simulink model "single_phase_thyristor_rect"  (R2022b)
settings: Solver=VariableStepAuto  StartTime=0.0  StopTime=0.04  RelTol=1e-3
undefined symbols (not defined in the file): p
libraries: spsThyristorLib x6, spsVoltageMeasurementLib x4, spsACVoltageSourceLib x3, spsCurrentMeasurementLib x1, spsMeanLib x1, spsSeriesRLCBranchLib x1, spspowerguiLib x1
settings Model: Creator=alman  LastModifiedBy=alman
settings SolverCC: ZeroCrossAlgorithm=Adaptive
settings DebuggingCC: MaskedZcDiagnostic=none  IgnoredZcDiagnostic=none

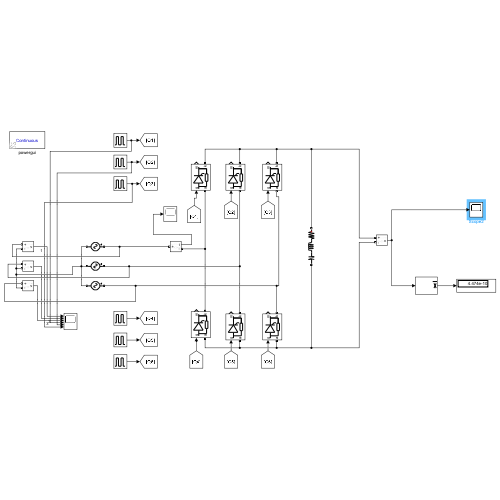
[thumbnail: Simulink's stored preview of the top-level diagram]
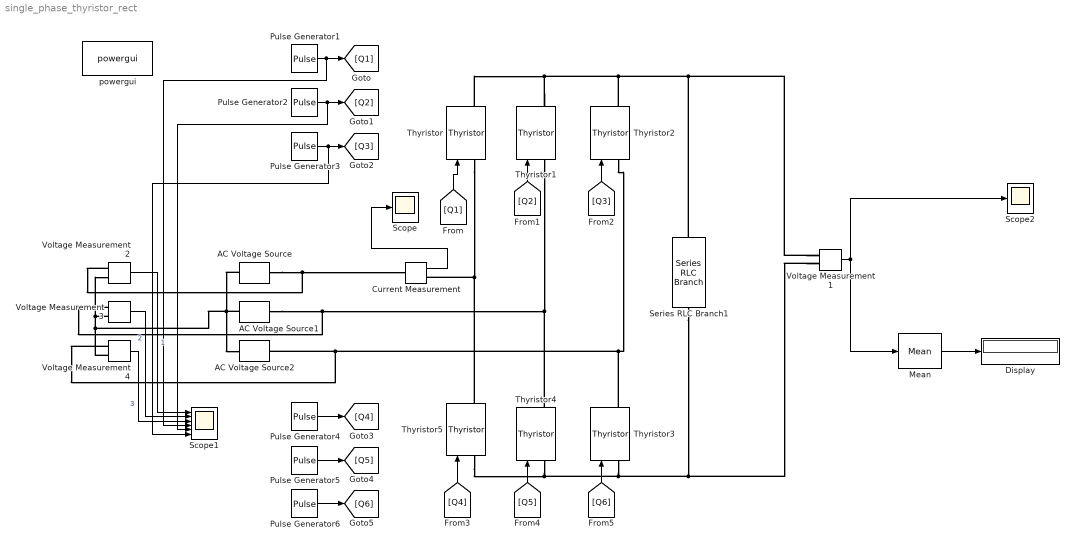
== system single_phase_thyristor_rect ==
  AC Voltage Source : spsACVoltageSourceLib/AC Voltage Source  Amplitude=230*sqrt(2)  Phase=0  Frequency=50  SampleTime=0  Measurements=None  BusType=swing  Pref=10e3  Qref=0  Qmin=-inf  Qmax=+inf
  AC Voltage Source1 : spsACVoltageSourceLib/AC Voltage Source  Amplitude=230*sqrt(2)  Phase=-120  Frequency=50  SampleTime=0  Measurements=None  BusType=swing  Pref=10e3  Qref=0  Qmin=-inf  Qmax=+inf
  AC Voltage Source2 : spsACVoltageSourceLib/AC Voltage Source  Amplitude=230*sqrt(2)  Phase=-240  Frequency=50  SampleTime=0  Measurements=None  BusType=swing  Pref=10e3  Qref=0  Qmin=-inf  Qmax=+inf
  Current Measurement : spsCurrentMeasurementLib/Current Measurement  PhasorSimulation=off  OutputType=Complex  PSBequivalent=0
  Display : Display
  Mean : spsMeanLib/Mean  Freq=300  Vinit=0  Ts=0
  Pulse Generator1 : DiscretePulseGenerator  PulseType=Time based  Amplitude=100  Period=1/50  PulseWidth=10  PhaseDelay=+(p-30)*(0.02/360)
  Pulse Generator2 : DiscretePulseGenerator  PulseType=Time based  Amplitude=100  Period=1/50  PulseWidth=10  PhaseDelay=-0.02*(2/3)+(p-30)*(0.02/360)
  Pulse Generator3 : DiscretePulseGenerator  PulseType=Time based  Amplitude=100  Period=1/50  PulseWidth=10  PhaseDelay=-0.02*(1/3)+(p-30)*(0.02/360)
  Pulse Generator4 : DiscretePulseGenerator  PulseType=Time based  Amplitude=100  Period=1/50  PulseWidth=10  PhaseDelay=-0.02*(1/3+1/6)+(p-30)*(0.02/360)
  Pulse Generator5 : DiscretePulseGenerator  PulseType=Time based  Amplitude=100  Period=1/50  PulseWidth=10  PhaseDelay=-0.02*(1+1/6)+(p-30)*(0.02/360)
  Pulse Generator6 : DiscretePulseGenerator  PulseType=Time based  Amplitude=100  Period=1/50  PulseWidth=10  PhaseDelay=-0.02*(2/3+1/6)+(p-30)*(0.02/360)
  Scope : Scope
  Scope1 : Scope  NumInputPorts=6
  Scope2 : Scope
  Series RLC Branch1 : spsSeriesRLCBranchLib/Series RLC Branch  LConnTagsString=__new0  RConnTagsString=__new0  BranchType=RLC  Resistance=1  Inductance=1e-3  SetiL0=off  InitialCurrent=0  Capacitance=1e-6  Setx0=off  InitialVoltage=0  Measurements=None
  Thyristor{,1..5} (6 alike) : spsThyristorLib/Thyristor  Ron=0.001  Lon=0  Vf=0.8  IC=0  Rs=500  Cs=250e-9  Measurements=on
  Voltage Measurement{1..4} (4 alike) : spsVoltageMeasurementLib/Voltage Measurement  PhasorSimulation=off  OutputType=Complex  PSBequivalent=0
  powergui : spspowerguiLib/powergui  Priority=1  SimulationMode=Continuous  SampleTime=50e-6  frequency=60  Iterations=50  frequencyindice=50  Pbase=100e6  ErrMax=1e-4  UnitsV=kV  UnitsW=MW  buscounter=0  FunctionMessages=off  echomessages=off  EnableUseOfTLC=off  CurrentSourceSwitches=off  DisableSnubberDevices=off  DisableRonSwitches=off  DisableVfSwitches=off  DisplayEquations=off  AutomaticDiscreteSolvers=off  SolverType=Tustin/Backward Euler (TBE)  Interpol=off  ExternalGateDelay=off  methode=off  Ts=100  x0status=blocks  SPID=on  SwTol=0  HookPort=off  NonlinearTolerance=1e-4  nMaxIteration=100  ContinueOnMaxIteration=off  RestoreLinks=warning  ResistiveCurrentMeasurement=off  Frange=[0:2:500]  Ylog=off  Xlog=on  ShowGrid=off  save=off  variable=ZData  structure=0  ZoomFFT=off  StartTime=0.0  cycles=1  DisplayStyle=1  fundamental=60  FreqAxis=off  MaxFrequency=1000  frequencyindicesteady=1  RmsSteady=1  display=off
  wires:
  Current Measurement/1 -> Scope/1
  Voltage Measurement1/1 -> Mean/1, Scope2/1
  Pulse Generator1/1 -> Scope1/4, [Q1]
  Pulse Generator2/1 -> Scope1/5, [Q2]
  Pulse Generator3/1 -> Scope1/6, [Q3]
  [Q1] -> Thyristor/1
  [Q4] -> Thyristor5/1
  [Q5] -> Thyristor4/1
  [Q6] -> Thyristor3/1
  Pulse Generator4/1 -> [Q4]
  Pulse Generator5/1 -> [Q5]
  Pulse Generator6/1 -> [Q6]
  [Q3] -> Thyristor2/1
  [Q2] -> Thyristor1/1
  Mean/1 -> Display/1
  Voltage Measurement2/1 -> Scope1/1  "1"
  Voltage Measurement3/1 -> Scope1/2  "2"
  Voltage Measurement4/1 -> Scope1/3  "3"
  connections:
  AC Voltage Source1/RConn1 -- Voltage Measurement3/LConn1 -- Thyristor1/LConn1 -- Thyristor4/RConn1
  Current Measurement/RConn1 -- Thyristor5/RConn1 -- Thyristor/LConn1
  Thyristor3/LConn1 -- Voltage Measurement1/LConn2 -- Series RLC Branch1/RConn1 -- Thyristor4/LConn1 -- Thyristor5/LConn1
  AC Voltage Source/RConn1 -- Voltage Measurement2/LConn1 -- Current Measurement/LConn1
  Thyristor3/RConn1 -- Voltage Measurement4/LConn1 -- AC Voltage Source2/RConn1 -- Thyristor2/LConn1
  Thyristor/RConn1 -- Thyristor1/RConn1 -- Voltage Measurement1/LConn1 -- Series RLC Branch1/LConn1 -- Thyristor2/RConn1
  AC Voltage Source/LConn1 -- Voltage Measurement2/LConn2 -- Voltage Measurement3/LConn2 -- Voltage Measurement4/LConn2 -- AC Voltage Source2/LConn1 -- AC Voltage Source1/LConn1
